simulink model "ADCINP"  (R2022b)
settings: configuration reference "SharedConfig" (kept outside this file)
values from neighbouring files (symbols this model uses):
  DT_ADCINP_C = 0.0001    [ADCINP.sldd]
  HvBusCurDialEna_C = 1.0    [ADCINP.sldd]
  HvBusCurDialVal_C = 0.0    [ADCINP.sldd]
  HvBusCurFilTiCon_C = 0.0    [ADCINP.sldd]
  HvBusCurGain_C = 0.001548    [ADCINP.sldd]
  HvBusCurOfs_C = 0.0    [ADCINP.sldd]
  HvBusUDialEna_C = 1.0    [ADCINP.sldd]
  HvBusUDialVal_C = 0.0    [ADCINP.sldd]
  HvBusUFilTiCon_C = 0.0    [ADCINP.sldd]
  HvBusUGain_C = 0.0152    [ADCINP.sldd]
  HvBusUOfs_C = 0.0    [ADCINP.sldd]
  PhaCurADialEna_C = 1.0    [ADCINP.sldd]
  PhaCurADialVal_C = 0.0    [ADCINP.sldd]
  PhaCurAFilTiCon_C = 0.0    [ADCINP.sldd]
  PhaCurAGain_C = 0.001548    [ADCINP.sldd]
  PhaCurAOfs_C = -3.06    [ADCINP.sldd]
  PhaCurBDialEna_C = 1.0    [ADCINP.sldd]
  PhaCurBDialVal_C = 0.0    [ADCINP.sldd]
  PhaCurBFilTiCon_C = 0.0    [ADCINP.sldd]
  PhaCurBGain_C = 0.001548    [ADCINP.sldd]
  PhaCurBOfs_C = -3.06    [ADCINP.sldd]
  PhaCurCDialEna_C = 1.0    [ADCINP.sldd]
  PhaCurCDialVal_C = 0.0    [ADCINP.sldd]
  PhaCurCFilTiCon_C = 0.0    [ADCINP.sldd]
  PhaCurCGain_C = 0.001548    [ADCINP.sldd]
  PhaCurCOfs_C = -3.06    [ADCINP.sldd]
  PhaUAFilTiCon_C = 0.0    [ADCINP.sldd]
  PhaUAGain_C = 0.0152    [ADCINP.sldd]
  PhaUAOfs_C = 0.0    [ADCINP.sldd]
  PhaUBFilTiCon_C = 0.0    [ADCINP.sldd]
  PhaUBGain_C = 0.0152    [ADCINP.sldd]
  PhaUBOfs_C = 0.0    [ADCINP.sldd]
  PhaUCFilTiCon_C = 0.0    [ADCINP.sldd]
  PhaUCGain_C = 0.0152    [ADCINP.sldd]
  PhaUCOfs_C = 0.0    [ADCINP.sldd]
  ResolverCosFilTiCon_C = 0.0    [ADCINP.sldd]
  ResolverCosGain_C = 0.0    [ADCINP.sldd]
  ResolverCosOfs_C = 0.0    [ADCINP.sldd]
  ResolverSinCosDialEna_C = 1.0    [ADCINP.sldd]
  ResolverSinCosDialVal_CA : value not decoded    [ADCINP.sldd]
  ResolverSinFilTiCon_C = 0.0    [ADCINP.sldd]
  ResolverSinGain_C = 0.0    [ADCINP.sldd]
  ResolverSinOfs_C = 0.0    [ADCINP.sldd]
undefined symbols (not defined in the file or in its folder): slcm
libraries: BlockLibrary x10
Description:
  | Converts raw analog inputs into engineering units.
settings Model: DataDictionary=ADCINP.sldd  Creator=Kevin  LastModifiedBy=Max Kolesnikov
settings ConfigSetRef: SourceName=SharedConfig

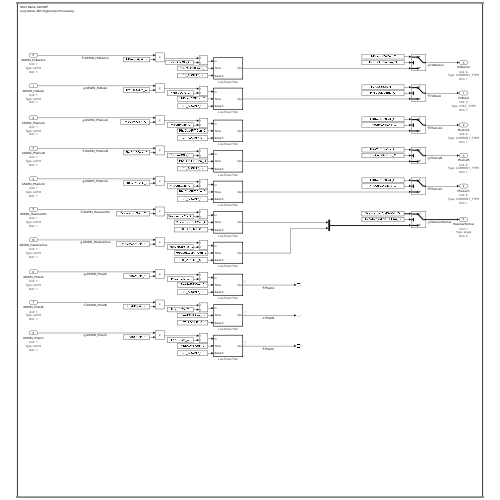
[thumbnail: Simulink's stored preview of the top-level diagram]
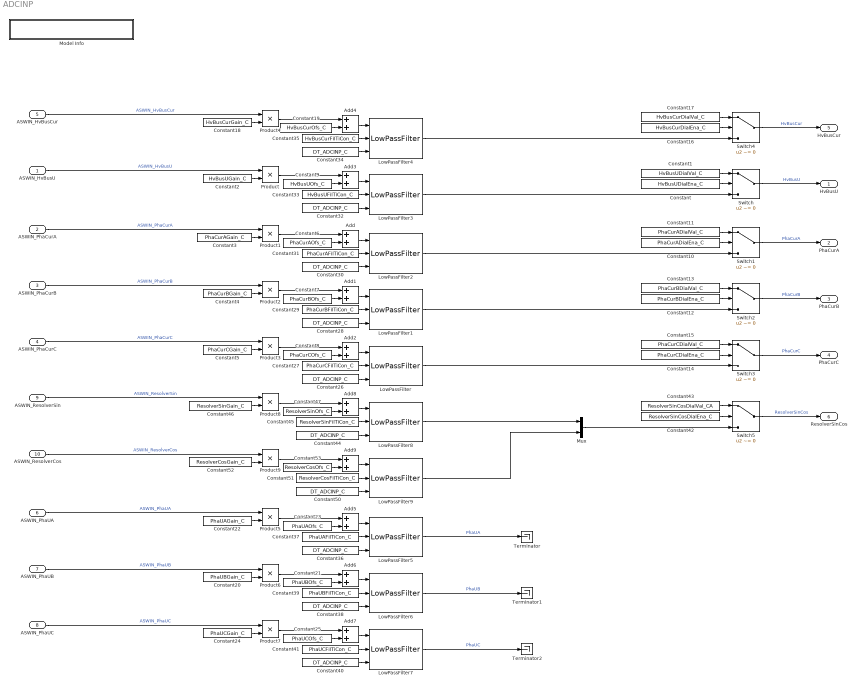
== system ADCINP ==
  ASWIN_HvBusU : Inport  OutDataTypeStr=uint16  Unit=1  PortDimensions=1
      settings: AttributesFormatString=|
      | Unit: %<Unit>
      | Type: %<OutDataTypeStr>
      | Dim: %<PortDimensions>
  ASWIN_PhaCurA : Inport  Port=2  OutDataTypeStr=uint16  Unit=1  PortDimensions=1
      settings: AttributesFormatString=|
      | Unit: %<Unit>
      | Type: %<OutDataTypeStr>
      | Dim: %<PortDimensions>
  ASWIN_PhaCurB : Inport  Port=3  OutDataTypeStr=uint16  Unit=1  PortDimensions=1
      settings: AttributesFormatString=|
      | Unit: %<Unit>
      | Type: %<OutDataTypeStr>
      | Dim: %<PortDimensions>
  ASWIN_PhaCurC : Inport  Port=4  OutDataTypeStr=uint16  Unit=1  PortDimensions=1
      settings: AttributesFormatString=|
      | Unit: %<Unit>
      | Type: %<OutDataTypeStr>
      | Dim: %<PortDimensions>
  ASWIN_HvBusCur : Inport  Port=5  OutDataTypeStr=uint16  Unit=1  PortDimensions=1
      settings: AttributesFormatString=|
      | Unit: %<Unit>
      | Type: %<OutDataTypeStr>
      | Dim: %<PortDimensions>
  ASWIN_PhaUA : Inport  Port=6  OutDataTypeStr=uint16  Unit=1  PortDimensions=1
      settings: AttributesFormatString=|
      | Unit: %<Unit>
      | Type: %<OutDataTypeStr>
      | Dim: %<PortDimensions>
  ASWIN_PhaUB : Inport  Port=7  OutDataTypeStr=uint16  Unit=1  PortDimensions=1
      settings: AttributesFormatString=|
      | Unit: %<Unit>
      | Type: %<OutDataTypeStr>
      | Dim: %<PortDimensions>
  ASWIN_PhaUC : Inport  Port=8  OutDataTypeStr=uint16  Unit=1  PortDimensions=1
      settings: AttributesFormatString=|
      | Unit: %<Unit>
      | Type: %<OutDataTypeStr>
      | Dim: %<PortDimensions>
  ASWIN_ResolverSin : Inport  Port=9  OutDataTypeStr=uint16  Unit=1  PortDimensions=1
      settings: AttributesFormatString=|
      | Unit: %<Unit>
      | Type: %<OutDataTypeStr>
      | Dim: %<PortDimensions>
  ASWIN_ResolverCos : Inport  Port=10  OutDataTypeStr=uint16  Unit=1  PortDimensions=1
      settings: AttributesFormatString=|
      | Unit: %<Unit>
      | Type: %<OutDataTypeStr>
      | Dim: %<PortDimensions>
  Add{,1..9} (10 alike) : Sum
  Constant : Constant  Value=HvBusUDialEna_C
  Constant1 : Constant  Value=HvBusUDialVal_C
  Constant10 : Constant  Value=PhaCurADialEna_C
  Constant11 : Constant  Value=PhaCurADialVal_C
  Constant12 : Constant  Value=PhaCurBDialEna_C
  Constant13 : Constant  Value=PhaCurBDialVal_C
  Constant14 : Constant  Value=PhaCurCDialEna_C
  Constant15 : Constant  Value=PhaCurCDialVal_C
  Constant16 : Constant  Value=HvBusCurDialEna_C
  Constant17 : Constant  Value=HvBusCurDialVal_C
  Constant18 : Constant  Value=HvBusCurGain_C
  Constant19 : Constant  Value=HvBusCurOfs_C
  Constant2 : Constant  Value=HvBusUGain_C
  Constant20 : Constant  Value=PhaUBGain_C
  Constant21 : Constant  Value=PhaUBOfs_C
  Constant22 : Constant  Value=PhaUAGain_C
  Constant23 : Constant  Value=PhaUAOfs_C
  Constant24 : Constant  Value=PhaUCGain_C
  Constant25 : Constant  Value=PhaUCOfs_C
  Constant{26,28,30,32,34,36,38,40,44,50} (10 alike) : Constant  Value=DT_ADCINP_C
  Constant27 : Constant  Value=PhaCurCFilTiCon_C
  Constant29 : Constant  Value=PhaCurBFilTiCon_C
  Constant3 : Constant  Value=PhaCurAGain_C
  Constant31 : Constant  Value=PhaCurAFilTiCon_C
  Constant33 : Constant  Value=HvBusUFilTiCon_C
  Constant35 : Constant  Value=HvBusCurFilTiCon_C
  Constant37 : Constant  Value=PhaUAFilTiCon_C
  Constant39 : Constant  Value=PhaUBFilTiCon_C
  Constant4 : Constant  Value=PhaCurBGain_C
  Constant41 : Constant  Value=PhaUCFilTiCon_C
  Constant42 : Constant  Value=ResolverSinCosDialEna_C
  Constant43 : Constant  Value=ResolverSinCosDialVal_CA
  Constant45 : Constant  Value=ResolverSinFilTiCon_C
  Constant46 : Constant  Value=ResolverSinGain_C
  Constant47 : Constant  Value=ResolverSinOfs_C
  Constant5 : Constant  Value=PhaCurCGain_C
  Constant51 : Constant  Value=ResolverCosFilTiCon_C
  Constant52 : Constant  Value=ResolverCosGain_C
  Constant53 : Constant  Value=ResolverCosOfs_C
  Constant6 : Constant  Value=PhaCurAOfs_C
  Constant7 : Constant  Value=PhaCurBOfs_C
  Constant8 : Constant  Value=PhaCurCOfs_C
  Constant9 : Constant  Value=HvBusUOfs_C
  LowPassFilter{,1..9} (10 alike) : BlockLibrary/LowPassFilter  Description=Low-Pass Filter  SystemSampleTime=-1  VariantActivationTime=update diagram  Latency=0  AutoFrameSizeCalculation=off
      settings: AttributesFormatString=%<Description>
  Model Info : Subsystem  LoadFcn=slcm LoadBlock;  InitFcn=slcm('UpdateAllCMBlocksInThisModelInit')  mask(CMBlock){Frame=off, DisplayStringWithTags=|, MaskDisplayString=Short Name: ADCINP\nLong Name: ADC Signal Input Processing, HorizontalTextAlignment=Left, LeftAlignmentValue=0.02}
      mask DisplayStringWithTags=|
      | Short Name: %<ModelName>
      | Long Name: ADC Signal Input Processing
      mask prompts: Frame "Simulink:masks:Frame_MP"; DisplayStringWithTags "Simulink:masks:DisplayStringWithTags_MP"; MaskDisplayString "Simulink:masks:MaskDisplayString_MP"; HorizontalTextAlignment "Simulink:masks:HorizontalTextAlignment_MP"; LeftAlignmentValue "Simulink:masks:LeftAlignmentValue_MP"
      mask help: Simulink:masks:CMBlock_MD
      settings: CopyFcn=slcm CopyBlock;  DeleteFcn=slcm Cancel;  PostSaveFcn=slcm('UpdateAllCMBlocksInThisModel')  NameChangeFcn=slcm Rename;  OpenFcn=slcm
      mask Display: text(slResolve(LeftAlignmentValue, gcbh), 0.5, MaskDisplayString, 'HorizontalAlignment', HorizontalTextAlignment)
  Mux : Mux  Inputs=2
  Product{,1..9} (10 alike) : Product
  Switch{,1..5} (6 alike) : Switch  Criteria=u2 ~= 0  SaturateOnIntegerOverflow=off  InputSameDT=off
  Terminator : Terminator
  Terminator1 : Terminator
  Terminator2 : Terminator
  HvBusU : Outport  OutDataTypeStr=VOLT_TYPE  Unit=V  PortDimensions=1
      settings: AttributesFormatString=|
      | Unit: %<Unit>
      | Type: %<OutDataTypeStr>
      | Dim: %<PortDimensions>
  PhaCurA : Outport  Port=2  OutDataTypeStr=CURRENT_TYPE  Unit=A  PortDimensions=1
      settings: AttributesFormatString=|
      | Unit: %<Unit>
      | Type: %<OutDataTypeStr>
      | Dim: %<PortDimensions>
  PhaCurB : Outport  Port=3  OutDataTypeStr=CURRENT_TYPE  Unit=A  PortDimensions=1
      settings: AttributesFormatString=|
      | Unit: %<Unit>
      | Type: %<OutDataTypeStr>
      | Dim: %<PortDimensions>
  PhaCurC : Outport  Port=4  OutDataTypeStr=CURRENT_TYPE  Unit=A  PortDimensions=1
      settings: AttributesFormatString=|
      | Unit: %<Unit>
      | Type: %<OutDataTypeStr>
      | Dim: %<PortDimensions>
  HvBusCur : Outport  Port=5  OutDataTypeStr=CURRENT_TYPE  Unit=A  PortDimensions=1
      settings: AttributesFormatString=|
      | Unit: %<Unit>
      | Type: %<OutDataTypeStr>
      | Dim: %<PortDimensions>
  ResolverSinCos : Outport  Port=6  OutDataTypeStr=single  Unit=1  PortDimensions=2
      settings: AttributesFormatString=|
      | Unit: %<Unit>
      | Type: %<OutDataTypeStr>
      | Dim: %<PortDimensions>
  wires:
  Constant1/1 -> Switch/1
  Constant/1 -> Switch/2
  Switch/1 -> HvBusU/1  "HvBusU"
  ASWIN_HvBusU/1 -> Product/1  "ASWIN_HvBusU"
  Switch1/1 -> PhaCurA/1  "PhaCurA"
  Constant2/1 -> Product/2
  Constant3/1 -> Product1/2
  ASWIN_PhaCurA/1 -> Product1/1  "ASWIN_PhaCurA"
  ASWIN_PhaCurB/1 -> Product2/1  "ASWIN_PhaCurB"
  Constant4/1 -> Product2/2
  Constant5/1 -> Product3/2
  ASWIN_PhaCurC/1 -> Product3/1  "ASWIN_PhaCurC"
  Constant6/1 -> Add/2
  Constant7/1 -> Add1/2
  Constant8/1 -> Add2/2
  Constant9/1 -> Add3/2
  Product1/1 -> Add/1
  Product2/1 -> Add1/1
  Product3/1 -> Add2/1
  Product/1 -> Add3/1
  Constant10/1 -> Switch1/2
  Constant11/1 -> Switch1/1
  Constant13/1 -> Switch2/1
  Constant12/1 -> Switch2/2
  Constant14/1 -> Switch3/2
  Constant15/1 -> Switch3/1
  Add2/1 -> LowPassFilter/1
  Switch2/1 -> PhaCurB/1  "PhaCurB"
  Switch3/1 -> PhaCurC/1  "PhaCurC"
  Constant17/1 -> Switch4/1
  Constant16/1 -> Switch4/2
  Product4/1 -> Add4/1
  Constant19/1 -> Add4/2
  ASWIN_HvBusCur/1 -> Product4/1  "ASWIN_HvBusCur"
  Constant18/1 -> Product4/2
  Switch4/1 -> HvBusCur/1  "HvBusCur"
  ASWIN_PhaUA/1 -> Product5/1  "ASWIN_PhaUA"
  Constant22/1 -> Product5/2
  Constant23/1 -> Add5/2
  Product5/1 -> Add5/1
  Product6/1 -> Add6/1
  Constant21/1 -> Add6/2
  Constant20/1 -> Product6/2
  ASWIN_PhaUB/1 -> Product6/1  "ASWIN_PhaUB"
  ASWIN_PhaUC/1 -> Product7/1  "ASWIN_PhaUC"
  Constant24/1 -> Product7/2
  Constant25/1 -> Add7/2
  Product7/1 -> Add7/1
  LowPassFilter/1 -> Switch3/3
  Constant26/1 -> LowPassFilter/3
  Constant27/1 -> LowPassFilter/2
  Constant29/1 -> LowPassFilter1/2
  Constant28/1 -> LowPassFilter1/3
  Add1/1 -> LowPassFilter1/1
  LowPassFilter1/1 -> Switch2/3
  Constant30/1 -> LowPassFilter2/3
  Constant31/1 -> LowPassFilter2/2
  Add/1 -> LowPassFilter2/1
  LowPassFilter2/1 -> Switch1/3
  Constant33/1 -> LowPassFilter3/2
  Constant32/1 -> LowPassFilter3/3
  Add3/1 -> LowPassFilter3/1
  LowPassFilter3/1 -> Switch/3
  Constant34/1 -> LowPassFilter4/3
  Constant35/1 -> LowPassFilter4/2
  Add4/1 -> LowPassFilter4/1
  LowPassFilter4/1 -> Switch4/3
  Constant37/1 -> LowPassFilter5/2
  Constant36/1 -> LowPassFilter5/3
  Add5/1 -> LowPassFilter5/1
  LowPassFilter5/1 -> Terminator/1  "PhaUA"
  LowPassFilter6/1 -> Terminator1/1  "PhaUB"
  Constant38/1 -> LowPassFilter6/3
  Constant39/1 -> LowPassFilter6/2
  Add6/1 -> LowPassFilter6/1
  Constant41/1 -> LowPassFilter7/2
  Constant40/1 -> LowPassFilter7/3
  LowPassFilter7/1 -> Terminator2/1  "PhaUC"
  Add7/1 -> LowPassFilter7/1
  Add8/1 -> LowPassFilter8/1
  Constant42/1 -> Switch5/2
  Constant43/1 -> Switch5/1
  Constant44/1 -> LowPassFilter8/3
  Mux/1 -> Switch5/3
  Product8/1 -> Add8/1
  Switch5/1 -> ResolverSinCos/1  "ResolverSinCos"
  Constant46/1 -> Product8/2
  ASWIN_ResolverSin/1 -> Product8/1  "ASWIN_ResolverSin"
  Constant45/1 -> LowPassFilter8/2
  Constant47/1 -> Add8/2
  Product9/1 -> Add9/1
  Constant50/1 -> LowPassFilter9/3
  Constant52/1 -> Product9/2
  ASWIN_ResolverCos/1 -> Product9/1  "ASWIN_ResolverCos"
  Add9/1 -> LowPassFilter9/1
  Constant51/1 -> LowPassFilter9/2
  Constant53/1 -> Add9/2
  LowPassFilter9/1 -> Mux/2
  LowPassFilter8/1 -> Mux/1

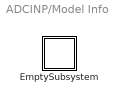
== system ADCINP/Model Info ==
  EmptySubsystem : Subsystem

== system ADCINP/Model Info/EmptySubsystem ==
